simulink model "MATE_Pejovic_inverter"  (R2024b)
settings: Solver=FixedStepDiscrete  StartTime=0.0  StopTime=0.01  FixedStep=Ts  RelTol=1e-3
PostLoadFcn:
  | Ts=1e-6
InitFcn:
  | Ts=1e-6
libraries: fl_lib x29, nesl_utility x14, simetranss x4, batteryecm_lib x3
settings Model: ARTEMISmethode_block_infos=$$__separator__$$  Creator=Kyle Diller  LastModifiedBy=CD8435
settings SolverCC: MaxOrder=2  AlgebraicLoopSolver=TrustRegion
settings DataIOCC: SaveFormat=Array  SignalLoggingSaveFormat=ModelDataLogs  ReturnWorkspaceOutputs=off  SignalLoggingName=sigsOut
settings OptimizationCC: BlockReduction=off  BooleanDataType=off  ExpressionDepthLimit=2147483647  InitFltsAndDblsToZero=on  LifeSpan=inf
settings DebuggingCC: SaveWithParameterizedLinksMsg=none  UnderspecifiedInitializationDetection=Classic  MergeDetectMultiDrivingBlocksExec=none  SignalResolutionControl=TryResolveAllWithWarning  MultiTaskDSMMsg=warning  MultiTaskCondExecSysMsg=none  FcnCallInpInsideContextMsg=warning  UnconnectedInputMsg=warning  UnconnectedOutputMsg=warning  UnconnectedLineMsg=warning  AllowSymbolicDim=off  StateNameClashWarn=warning  SFUnexpectedBacktrackingDiag=warning  SFNoUnconditionalDefaultTransitionDiag=warning  SFExecutionAtInitializationDiag=none  ArithmeticOperatorsInVariantConditions=warning
settings HardwareCC: ProdBitPerPointer=32  ProdBitPerSizeT=32  ProdBitPerPtrDiffT=32  ProdLargestAtomicFloat=None  ProdIntDivRoundTo=Undefined  ProdEndianess=Unspecified  ProdWordSize=32  ProdHWDeviceType=32-bit Generic  TargetUnknown=on
settings ModelReferenceCC: EnableRefExpFcnMdlSchedulingChecks=on  PropagateSignalLabelsOutOfModel=off
settings SFSimCC: SimUseLocalCustomCode=off  CustomCodeUndefinedFunction=UseInterfaceOnly
settings RTWCC: TemplateMakefile=grt_unix.tmf  RTWUseLocalCustomCode=off  GPUComputeCapability=3.5
settings CodeAppCC: StateflowObjectComments=on
settings GRTTargetCC: TargetFcnLib=ansi_tfl_tmw.mat  TargetLangStandard=C89/C90 (ANSI)  CombineOutputUpdateFcns=off  GRTInterface=on
settings ConfigComp: CovMetricSettings=dw  CovSaveCumulativeToWorkspaceVar=on  CovSaveSingleToWorkspaceVar=on  CovExternalEMLEnable=off
settings SimscapeCC: SimscapeNormalizeSystem=off

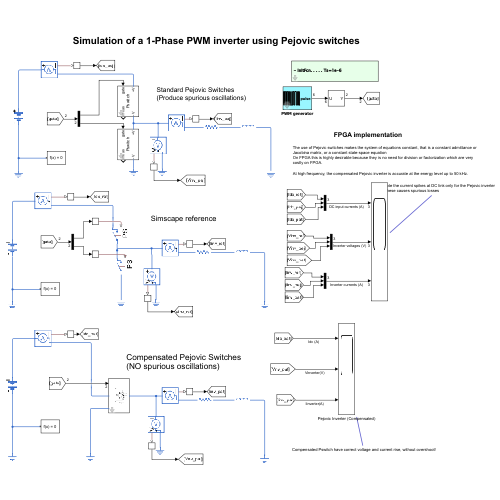
[thumbnail: Simulink's stored preview of the top-level diagram]
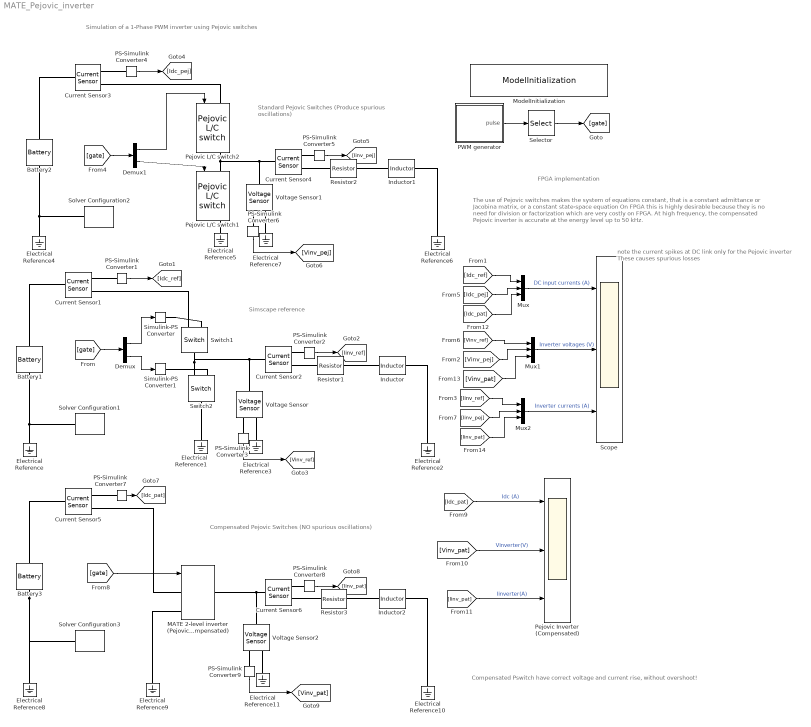
== system MATE_Pejovic_inverter ==
  note: The use of Pejovic switches makes the system of equations constant, that is a constant admittance or Jacobina matrix, or a constant state-space equation
      | On FPGA this is highly desirable because they is no need for division or factorization which are very costly on FPGA.
      |
      | At high frequency, the compensated Pejovic inverter is accurate at the energy level up to 50 kHz.
  note: FPGA implementation
  note: Simscape reference
  note: Standard Pejovic Switches
      | (Produce spurious oscillations)
  note: Compensated Pswitch have correct voltage and current rise, without overshoot!
  note: note the current spikes at DC link only for the Pejovic inverter
      | These causes spurious losses
  note: Simulation of a 1-Phase PWM inverter using Pejovic switches
  note: Compensated Pejovic Switches
      | (NO spurious oscillations)
  Battery1 : batteryecm_lib/Battery  Vnom=100 V  prm_dir=simscape.enum.battery.prm_dir.disabled  R1_dis=2 Ohm  R1_ch=2 Ohm  R1=0.5 Ohm  prm_AH=simscape.enum.battery.prm_AH.infinite  AH=50 A*hr  V1=11.5 V  AH1=25 A*hr  prm_R2=simscape.enum.battery.prm_R2.disabled  R2=2000 Ohm  Tmeas=298.15 K  charge_measurement_port=simscape.enum.battery.enable.no  prm_dyn=simscape.enum.battery.prm_dyn.off  Rp1=0.005 Ohm  tau1=30 s  Rp2=0.005 Ohm  tau2=30 s  Rp3=0.005 Ohm  tau3=30 s  Rp4=0.005 Ohm  tau4=30 s  Rp5=0.005 Ohm  tau5=30 s  prm_fade=simscape.enum.battery.prm_fade.disabled  N_fade=100  AH_fade=45 A*hr  R1_fade=2.02 Ohm  R1_ch_fade=2.02 Ohm  V1_fade=10.35 V  prm_age=simscape.enum.battery.prm_age.disabled  prm_age_OCV=simscape.enum.battery.prm_age_OCV.OCV  OCV_age=0.9  SOC_age=60  Tmeas_age=298.15 K  delta_time_age_vec=[0] d  temperature_age_vec=[273] K  OCV_scaling_age=2.2134e6  OCV_offset_age=1.632e6  temp_exp_age=0.515833569 V  t_exp_age=0.75  Vnom_T2=12 V  R1_T2=2.2 Ohm  R1_T2_dis=2.2 Ohm  R1_T2_ch=2.2 Ohm  V1_T2=11.4 V  R2_T2=2200 Ohm  Rp1_T2=0.005 Ohm  tau1_T2=30 s  Rp2_T2=0.005 Ohm  tau2_T2=30 s  Rp3_T2=0.005 Ohm  tau3_T2=30 s  Rp4_T2=0.005 Ohm  tau4_T2=30 s  Rp5_T2=0.005 Ohm  tau5_T2=30 s  Tmeas2=273.15 K  thermal_port=simscape.enum.thermaleffects.omit  thermal_mass=30000 J/K  i_specify=off  i_priority=None  i=0 A  i_nominal_specify=off  i_nominal_value=1  i_nominal_unit=A  v_specify=off  v_priority=None  v=0 V  v_nominal_specify=off  v_nominal_value=1  v_nominal_unit=V  charge_specify=off  charge_priority=High  charge=50 A*hr  charge_nominal_specify=off  charge_nominal_value=1  charge_nominal_unit=A*hr  num_cycles_specify=off  num_cycles_priority=High  num_cycles=0  num_cycles_nominal_specify=off  num_cycles_nominal_value=1  num_cycles_nominal_unit=1  temperature_specify=off  temperature_priority=High  temperature=298.15 K  temperature_nominal_specify=off  temperature_nominal_value=1  temperature_nominal_unit=K
  Battery2 : batteryecm_lib/Battery  Vnom=100 V  prm_dir=simscape.enum.battery.prm_dir.disabled  R1_dis=2 Ohm  R1_ch=2 Ohm  R1=0.5 Ohm  prm_AH=simscape.enum.battery.prm_AH.infinite  AH=50 A*hr  V1=11.5 V  AH1=25 A*hr  prm_R2=simscape.enum.battery.prm_R2.disabled  R2=2000 Ohm  Tmeas=298.15 K  charge_measurement_port=simscape.enum.battery.enable.no  prm_dyn=simscape.enum.battery.prm_dyn.off  Rp1=0.005 Ohm  tau1=30 s  Rp2=0.005 Ohm  tau2=30 s  Rp3=0.005 Ohm  tau3=30 s  Rp4=0.005 Ohm  tau4=30 s  Rp5=0.005 Ohm  tau5=30 s  prm_fade=simscape.enum.battery.prm_fade.disabled  N_fade=100  AH_fade=45 A*hr  R1_fade=2.02 Ohm  R1_ch_fade=2.02 Ohm  V1_fade=10.35 V  prm_age=simscape.enum.battery.prm_age.disabled  prm_age_OCV=simscape.enum.battery.prm_age_OCV.OCV  OCV_age=0.9  SOC_age=60  Tmeas_age=298.15 K  delta_time_age_vec=[0] d  temperature_age_vec=[273] K  OCV_scaling_age=2.2134e6  OCV_offset_age=1.632e6  temp_exp_age=0.515833569 V  t_exp_age=0.75  Vnom_T2=12 V  R1_T2=2.2 Ohm  R1_T2_dis=2.2 Ohm  R1_T2_ch=2.2 Ohm  V1_T2=11.4 V  R2_T2=2200 Ohm  Rp1_T2=0.005 Ohm  tau1_T2=30 s  Rp2_T2=0.005 Ohm  tau2_T2=30 s  Rp3_T2=0.005 Ohm  tau3_T2=30 s  Rp4_T2=0.005 Ohm  tau4_T2=30 s  Rp5_T2=0.005 Ohm  tau5_T2=30 s  Tmeas2=273.15 K  thermal_port=simscape.enum.thermaleffects.omit  thermal_mass=30000 J/K  i_specify=off  i_priority=None  i=0 A  i_nominal_specify=off  i_nominal_value=1  i_nominal_unit=A  v_specify=off  v_priority=None  v=0 V  v_nominal_specify=off  v_nominal_value=1  v_nominal_unit=V  charge_specify=off  charge_priority=High  charge=50 A*hr  charge_nominal_specify=off  charge_nominal_value=1  charge_nominal_unit=A*hr  num_cycles_specify=off  num_cycles_priority=High  num_cycles=0  num_cycles_nominal_specify=off  num_cycles_nominal_value=1  num_cycles_nominal_unit=1  temperature_specify=off  temperature_priority=High  temperature=298.15 K  temperature_nominal_specify=off  temperature_nominal_value=1  temperature_nominal_unit=K
  Battery3 : batteryecm_lib/Battery  Vnom=100 V  prm_dir=simscape.enum.battery.prm_dir.disabled  R1_dis=2 Ohm  R1_ch=2 Ohm  R1=0.5 Ohm  prm_AH=simscape.enum.battery.prm_AH.infinite  AH=50 A*hr  V1=11.5 V  AH1=25 A*hr  prm_R2=simscape.enum.battery.prm_R2.disabled  R2=2000 Ohm  Tmeas=298.15 K  charge_measurement_port=simscape.enum.battery.enable.no  prm_dyn=simscape.enum.battery.prm_dyn.off  Rp1=0.005 Ohm  tau1=30 s  Rp2=0.005 Ohm  tau2=30 s  Rp3=0.005 Ohm  tau3=30 s  Rp4=0.005 Ohm  tau4=30 s  Rp5=0.005 Ohm  tau5=30 s  prm_fade=simscape.enum.battery.prm_fade.disabled  N_fade=100  AH_fade=45 A*hr  R1_fade=2.02 Ohm  R1_ch_fade=2.02 Ohm  V1_fade=10.35 V  prm_age=simscape.enum.battery.prm_age.disabled  prm_age_OCV=simscape.enum.battery.prm_age_OCV.OCV  OCV_age=0.9  SOC_age=60  Tmeas_age=298.15 K  delta_time_age_vec=[0] d  temperature_age_vec=[273] K  OCV_scaling_age=2.2134e6  OCV_offset_age=1.632e6  temp_exp_age=0.515833569 V  t_exp_age=0.75  Vnom_T2=12 V  R1_T2=2.2 Ohm  R1_T2_dis=2.2 Ohm  R1_T2_ch=2.2 Ohm  V1_T2=11.4 V  R2_T2=2200 Ohm  Rp1_T2=0.005 Ohm  tau1_T2=30 s  Rp2_T2=0.005 Ohm  tau2_T2=30 s  Rp3_T2=0.005 Ohm  tau3_T2=30 s  Rp4_T2=0.005 Ohm  tau4_T2=30 s  Rp5_T2=0.005 Ohm  tau5_T2=30 s  Tmeas2=273.15 K  thermal_port=simscape.enum.thermaleffects.omit  thermal_mass=30000 J/K  i_specify=off  i_priority=None  i=0 A  i_nominal_specify=off  i_nominal_value=1  i_nominal_unit=A  v_specify=off  v_priority=None  v=0 V  v_nominal_specify=off  v_nominal_value=1  v_nominal_unit=V  charge_specify=off  charge_priority=High  charge=50 A*hr  charge_nominal_specify=off  charge_nominal_value=1  charge_nominal_unit=A*hr  num_cycles_specify=off  num_cycles_priority=High  num_cycles=0  num_cycles_nominal_specify=off  num_cycles_nominal_value=1  num_cycles_nominal_unit=1  temperature_specify=off  temperature_priority=High  temperature=298.15 K  temperature_nominal_specify=off  temperature_nominal_value=1  temperature_nominal_unit=K
  Current Sensor{1..6} (6 alike) : fl_lib/Electrical/Electrical Sensors/Current Sensor
  Demux : Demux  Outputs=2
  Demux1 : Demux  Outputs=2
  Electrical Reference{,1..11} (12 alike) : fl_lib/Electrical/Electrical Elements/Electrical Reference
  Inductor : fl_lib/Electrical/Electrical Elements/Inductor  l=1e-4 H  r=0 Ohm  g=1e-9 1/Ohm  i_specify=off  i_priority=None  i=0 A  i_nominal_specify=off  i_nominal_value=1  i_nominal_unit=A  v_specify=off  v_priority=None  v=0 V  v_nominal_specify=off  v_nominal_value=1  v_nominal_unit=V  i_L_specify=off  i_L_priority=High  i_L=0 A  i_L_nominal_specify=off  i_L_nominal_value=1  i_L_nominal_unit=A
  Inductor1 : fl_lib/Electrical/Electrical Elements/Inductor  l=1e-4 H  r=0 Ohm  g=1e-9 1/Ohm  i_specify=off  i_priority=None  i=0 A  i_nominal_specify=off  i_nominal_value=1  i_nominal_unit=A  v_specify=off  v_priority=None  v=0 V  v_nominal_specify=off  v_nominal_value=1  v_nominal_unit=V  i_L_specify=off  i_L_priority=High  i_L=0 A  i_L_nominal_specify=off  i_L_nominal_value=1  i_L_nominal_unit=A
  Inductor2 : fl_lib/Electrical/Electrical Elements/Inductor  l=1e-4 H  r=0 Ohm  g=1e-9 1/Ohm  i_specify=off  i_priority=None  i=0 A  i_nominal_specify=off  i_nominal_value=1  i_nominal_unit=A  v_specify=off  v_priority=None  v=0 V  v_nominal_specify=off  v_nominal_value=1  v_nominal_unit=V  i_L_specify=off  i_L_priority=High  i_L=0 A  i_L_nominal_specify=off  i_L_nominal_value=1  i_L_nominal_unit=A
  MATE 2-level inverter (Pejovic Energy compensated) : simetranss/FPGA/MATE 2-level inverter (Pejovic Energy compensated)  Lon=1e-6  Ts=Ts
  ModelInitialization : simetranss/Usefulls/ModelInitialization  InitFcnX=Ts=1e-6  prel=off  posl=on  inif=on  strf=off
  Mux : Mux  Inputs=3
  Mux1 : Mux  Inputs=3
  Mux2 : Mux  Inputs=3
  PS-Simulink Converter{1..9} (9 alike) : nesl_utility/PS-Simulink Converter  PhysicalDomain=network_engine_domain  SubClassName=ps_output  LeftPortType=input  RightPortType=output  PseudoPeriodic=off  Frequencies=[]  VectorFormat=inherit  Unit=inherit  AffineConversion=off
  PWM generator : Subsystem  Tag=RTEcontrol_s38shd7k88  mask(3-phase Discrete PWM Generator){Fc=1080, Ts=Ts, mIndex=0.6, Freq=60, Phase=0}
      mask prompts: Fc "Carrier frequency (Hz):"; Ts "Sample time:"; mIndex "Modulation index  (0<m<1) :"; Freq "Frequency of output voltage (Hz)"; Phase "Phase of output voltage (degrees)"
      mask help: This block generates pulses for 3-phase carrier-based PWM (Pulse Width Modulation), self-commutated IGBTs,GTOs or FETs bridges in Simscape.
      mask init:
      | if Freq==0
      |     Phase=90;
      | end
      |     Internal_Phase=[0 -2*pi/3 2*pi/3];
      |     Signal_PortWidth=3;
      |     Select1_Elements=[1 4 2 5 3 6];
      |     Select1_PortWidth=6;
      |    Select3_Elements=[1 2 3 4 5 6];
      |    Select3_PortWidth=12;
      mask Display: plot(0,0,100,100,[60,57,57,56,56,53,53,50,50,47,47,41,41,38,38,35,35,32,32,31,31,25,25,24,24,22,22,19,19,16,16,11,11,8,8,5,5,3,3,2,2,0],[20,20,80,80,20,20,80,80,20,20,80,80,20,20,80,80,20,20,80,80,20,20,80,80,20,20,80,80,20,20,80,80,20,20,80,80,20,20,80,80,20,20])
  Pejovic Inverter (Compensated) : Scope  NumInputPorts=3
  Pejovic L/C switch1 : simetranss/FPGA/Pejovic L//C switch  Lon=1e-6  Ts=Ts
  Pejovic L/C switch2 : simetranss/FPGA/Pejovic L//C switch  Lon=1e-6  Ts=Ts
  Resistor1 : fl_lib/Electrical/Electrical Elements/Resistor  R=9.5 Ohm  i_specify=off  i_priority=None  i=0 A  i_nominal_specify=off  i_nominal_value=1  i_nominal_unit=A  v_specify=off  v_priority=None  v=0 V  v_nominal_specify=off  v_nominal_value=1  v_nominal_unit=V
  Resistor2 : fl_lib/Electrical/Electrical Elements/Resistor  R=9.5 Ohm  i_specify=off  i_priority=None  i=0 A  i_nominal_specify=off  i_nominal_value=1  i_nominal_unit=A  v_specify=off  v_priority=None  v=0 V  v_nominal_specify=off  v_nominal_value=1  v_nominal_unit=V
  Resistor3 : fl_lib/Electrical/Electrical Elements/Resistor  R=9.5 Ohm  i_specify=off  i_priority=None  i=0 A  i_nominal_specify=off  i_nominal_value=1  i_nominal_unit=A  v_specify=off  v_priority=None  v=0 V  v_nominal_specify=off  v_nominal_value=1  v_nominal_unit=V
  Scope : Scope  NumInputPorts=3
  Selector : Selector  InputPortWidth=6  IndexOptions=Index vector (dialog)  Indices=[1 2]  OutputSizes=1
  Simulink-PS Converter : nesl_utility/Simulink-PS Converter  PhysicalDomain=network_engine_domain  SubClassName=ps_input  LeftPortType=input  RightPortType=output  PseudoPeriodic=off  Frequencies=[]  NoiseDistribution=none  NoiseParameters=[]  Unit=1  AffineConversion=off  FilteringAndDerivatives=provide  SimscapeFilterOrder=1  InputFilterTimeConstant=0.001  UdotUserProvided=0
  Simulink-PS Converter1 : nesl_utility/Simulink-PS Converter  PhysicalDomain=network_engine_domain  SubClassName=ps_input  LeftPortType=input  RightPortType=output  PseudoPeriodic=off  Frequencies=[]  NoiseDistribution=none  NoiseParameters=[]  Unit=1  AffineConversion=off  FilteringAndDerivatives=provide  SimscapeFilterOrder=1  InputFilterTimeConstant=0.001  UdotUserProvided=0
  Solver Configuration1 : nesl_utility/Solver Configuration  PhysicalDomain=network_engine_domain  SubClassName=solver  LeftPortType=input  RightPortType=generic  Tones=[]  Harmonics=[]  SimulateNoise=off  Profile=off  UseLocalSampling=off  EnableSwitchedLinearOptims=on  FrequencyDomain=off  UseCCode=off  RelTol=0.001  AbsTol=0.001  MinStep=1e-09  ToWorkspace=off  RevertToSquareIcSolve=off  NumHomotopyIterations=100  PhasorMode=off  PhasorModeNumHarmonics=1  ConsistencySolver=NEWTON_XTOL_AFTER_FTOL  IndexReductionMethod=DerivativeReplacement  DoDC=off  ResidualTolerance=1e-09  ConsistencyTolSource=GLOBAL  ConsistencyAbsTol=0.001  ConsistencyRelTol=0.001  ConsistencyTolFactor=0.001  UseLocalSolver=on  LocalSolverChoice=NE_PARTITIONING_ADVANCER  ResolveIndetEquations=on  FunctionEvalNumThread=1  LocalSolverSampleTime=Ts  DoFixedCost=on  MaxNonlinIter=1  MaxModeIter=2  ComputeImpulses=off  ImpulseIterations=2  LinearAlgebra=auto  LinearAlgebraNumThread=0  EquationFormulation=NE_TIME_EF  DelaysMemoryBudget=1024  AutomaticFiltering=on  FilteringTimeConstant=0.001  PartitionStorageMethod=AS_NEEDED  PartitionMemoryBudget=1024  PartitionMethod=ROBUST  MultibodyUseLocalSolver=off  MultibodyLocalSolverChoice=ODE1  MultibodyLocalSolverSampleTime=0.001
  Solver Configuration2 : nesl_utility/Solver Configuration  PhysicalDomain=network_engine_domain  SubClassName=solver  LeftPortType=input  RightPortType=generic  Tones=[]  Harmonics=[]  SimulateNoise=off  Profile=off  UseLocalSampling=off  EnableSwitchedLinearOptims=on  FrequencyDomain=off  UseCCode=off  RelTol=0.001  AbsTol=0.001  MinStep=1e-09  ToWorkspace=off  RevertToSquareIcSolve=off  NumHomotopyIterations=100  PhasorMode=off  PhasorModeNumHarmonics=1  ConsistencySolver=NEWTON_XTOL_AFTER_FTOL  IndexReductionMethod=DerivativeReplacement  DoDC=off  ResidualTolerance=1e-09  ConsistencyTolSource=GLOBAL  ConsistencyAbsTol=0.001  ConsistencyRelTol=0.001  ConsistencyTolFactor=0.001  UseLocalSolver=on  LocalSolverChoice=NE_BACKWARD_EULER_ADVANCER  ResolveIndetEquations=on  FunctionEvalNumThread=1  LocalSolverSampleTime=Ts  DoFixedCost=on  MaxNonlinIter=1  MaxModeIter=2  ComputeImpulses=off  ImpulseIterations=2  LinearAlgebra=auto  LinearAlgebraNumThread=0  EquationFormulation=NE_TIME_EF  DelaysMemoryBudget=1024  AutomaticFiltering=on  FilteringTimeConstant=0.001  PartitionStorageMethod=AS_NEEDED  PartitionMemoryBudget=1024  PartitionMethod=ROBUST  MultibodyUseLocalSolver=off  MultibodyLocalSolverChoice=ODE1  MultibodyLocalSolverSampleTime=0.001
  Solver Configuration3 : nesl_utility/Solver Configuration  PhysicalDomain=network_engine_domain  SubClassName=solver  LeftPortType=input  RightPortType=generic  Tones=[]  Harmonics=[]  SimulateNoise=off  Profile=off  UseLocalSampling=off  EnableSwitchedLinearOptims=on  FrequencyDomain=off  UseCCode=off  RelTol=0.001  AbsTol=0.001  MinStep=1e-09  ToWorkspace=off  RevertToSquareIcSolve=off  NumHomotopyIterations=100  PhasorMode=off  PhasorModeNumHarmonics=1  ConsistencySolver=NEWTON_XTOL_AFTER_FTOL  IndexReductionMethod=DerivativeReplacement  DoDC=off  ResidualTolerance=1e-09  ConsistencyTolSource=GLOBAL  ConsistencyAbsTol=0.001  ConsistencyRelTol=0.001  ConsistencyTolFactor=0.001  UseLocalSolver=on  LocalSolverChoice=NE_BACKWARD_EULER_ADVANCER  ResolveIndetEquations=on  FunctionEvalNumThread=1  LocalSolverSampleTime=Ts  DoFixedCost=on  MaxNonlinIter=1  MaxModeIter=2  ComputeImpulses=off  ImpulseIterations=2  LinearAlgebra=auto  LinearAlgebraNumThread=0  EquationFormulation=NE_TIME_EF  DelaysMemoryBudget=1024  AutomaticFiltering=on  FilteringTimeConstant=0.001  PartitionStorageMethod=AS_NEEDED  PartitionMemoryBudget=1024  PartitionMethod=ROBUST  MultibodyUseLocalSolver=off  MultibodyLocalSolverChoice=ODE1  MultibodyLocalSolverSampleTime=0.001
  Switch1 : fl_lib/Electrical/Electrical Elements/Switch  R_closed=0.001 Ohm  G_open=1e-8 1/Ohm  Threshold=0.5  i_specify=off  i_priority=None  i=0 A  i_nominal_specify=off  i_nominal_value=1  i_nominal_unit=A  v_specify=off  v_priority=None  v=0 V  v_nominal_specify=off  v_nominal_value=1  v_nominal_unit=V
  Switch2 : fl_lib/Electrical/Electrical Elements/Switch  R_closed=0.001 Ohm  G_open=1e-8 1/Ohm  Threshold=0.5  i_specify=off  i_priority=None  i=0 A  i_nominal_specify=off  i_nominal_value=1  i_nominal_unit=A  v_specify=off  v_priority=None  v=0 V  v_nominal_specify=off  v_nominal_value=1  v_nominal_unit=V
  Voltage Sensor : fl_lib/Electrical/Electrical Sensors/Voltage Sensor
  Voltage Sensor1 : fl_lib/Electrical/Electrical Sensors/Voltage Sensor
  Voltage Sensor2 : fl_lib/Electrical/Electrical Sensors/Voltage Sensor
  wires:
  PWM generator/1(pulse) -> Selector/1
  Demux/1 -> Simulink-PS Converter/1
  Demux/2 -> Simulink-PS Converter1/1
  Selector/1 -> [gate]
  [gate] -> Demux/1
  PS-Simulink Converter1/1 -> [Idc_ref]
  PS-Simulink Converter2/1 -> [Iinv_ref]
  PS-Simulink Converter3/1 -> [Vinv_ref]
  PS-Simulink Converter6/1 -> [Vinv_pej]
  PS-Simulink Converter5/1 -> [Iinv_pej]
  PS-Simulink Converter4/1 -> [Idc_pej]
  [gate] -> Demux1/1
  Demux1/1 -> Pejovic L/C switch2/1
  Demux1/2 -> Pejovic L/C switch1/1
  Mux/1 -> Scope/1  "DC input currents (A)"
  [Idc_pej] -> Mux/2
  [Idc_ref] -> Mux/1
  [Vinv_pej] -> Mux1/2
  Mux1/1 -> Scope/2  "Inverter voltages (V)"
  [Vinv_ref] -> Mux1/1
  Mux2/1 -> Scope/3  "Inverter currents (A)"
  [Iinv_ref] -> Mux2/1
  [Iinv_pej] -> Mux2/2
  PS-Simulink Converter7/1 -> [Idc_pat]
  PS-Simulink Converter8/1 -> [Iinv_pat]
  PS-Simulink Converter9/1 -> [Vinv_pat]
  [Idc_pat] -> Pejovic Inverter (Compensated)/1  "Idc (A)"
  [Vinv_pat] -> Pejovic Inverter (Compensated)/2  "Vinverter(V)"
  [Iinv_pat] -> Pejovic Inverter (Compensated)/3  "Iinverter(A)"
  [Idc_pat] -> Mux/3
  [Vinv_pat] -> Mux1/3
  [Iinv_pat] -> Mux2/3
  [gate] -> MATE 2-level inverter (Pejovic Energy compensated)/1
  connections:
  Electrical Reference/LConn1 -- Solver Configuration1/RConn1 -- Battery1/RConn1
  Battery1/LConn1 -- Current Sensor1/LConn1
  Current Sensor1/RConn2 -- Switch1/RConn2
  Switch2/RConn2 -- Voltage Sensor/LConn1 -- Current Sensor2/LConn1 -- Switch1/LConn1
  Electrical Reference1/LConn1 -- Switch2/LConn1
  Inductor/LConn1 -- Resistor1/RConn1
  Inductor/RConn1 -- Electrical Reference2/LConn1
  Current Sensor2/RConn2 -- Resistor1/LConn1
  PS-Simulink Converter1/LConn1 -- Current Sensor1/RConn1
  PS-Simulink Converter2/LConn1 -- Current Sensor2/RConn1
  Electrical Reference3/LConn1 -- Voltage Sensor/RConn2
  PS-Simulink Converter3/LConn1 -- Voltage Sensor/RConn1
  Simulink-PS Converter/RConn1 -- Switch1/RConn1
  Simulink-PS Converter1/RConn1 -- Switch2/RConn1
  Electrical Reference4/LConn1 -- Battery2/RConn1 -- Solver Configuration2/RConn1
  PS-Simulink Converter6/LConn1 -- Voltage Sensor1/RConn1
  Electrical Reference7/LConn1 -- Voltage Sensor1/RConn2
  PS-Simulink Converter5/LConn1 -- Current Sensor4/RConn1
  PS-Simulink Converter4/LConn1 -- Current Sensor3/RConn1
  Inductor1/LConn1 -- Resistor2/RConn1
  Current Sensor4/RConn2 -- Resistor2/LConn1
  Inductor1/RConn1 -- Electrical Reference6/LConn1
  Battery2/LConn1 -- Current Sensor3/LConn1
  Pejovic L/C switch2/LConn1 -- Current Sensor3/RConn2
  Current Sensor4/LConn1 -- Pejovic L/C switch1/LConn1 -- Pejovic L/C switch2/RConn1 -- Voltage Sensor1/LConn1
  Pejovic L/C switch1/RConn1 -- Electrical Reference5/LConn1
  Battery3/RConn1 -- Electrical Reference8/LConn1 -- Solver Configuration3/RConn1
  Current Sensor6/LConn1 -- MATE 2-level inverter (Pejovic Energy compensated)/RConn1 -- Voltage Sensor2/LConn1
  Battery3/LConn1 -- Current Sensor5/LConn1
  Inductor2/RConn1 -- Electrical Reference10/LConn1
  Current Sensor6/RConn2 -- Resistor3/LConn1
  Electrical Reference11/LConn1 -- Voltage Sensor2/RConn2
  PS-Simulink Converter8/LConn1 -- Current Sensor6/RConn1
  PS-Simulink Converter7/LConn1 -- Current Sensor5/RConn1
  PS-Simulink Converter9/LConn1 -- Voltage Sensor2/RConn1
  Inductor2/LConn1 -- Resistor3/RConn1
  MATE 2-level inverter (Pejovic Energy compensated)/LConn1 -- Current Sensor5/RConn2
  MATE 2-level inverter (Pejovic Energy compensated)/LConn2 -- Electrical Reference9/LConn1

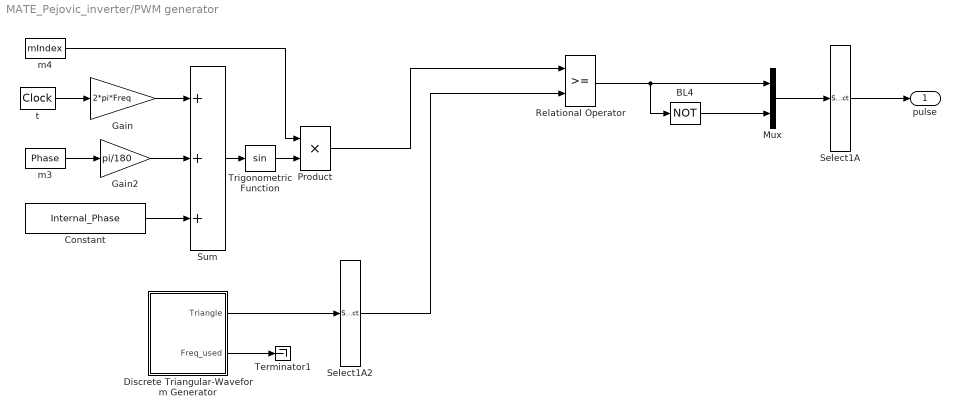
== system MATE_Pejovic_inverter/PWM generator ==
  BL4 : Logic  Operator=NOT  Inputs=1
  Constant : Constant  Value=Internal_Phase
  Discrete Triangular-Waveform Generator : Subsystem  mask(Discrete Triangular-Waveform  Generator){Freq=Fc, Vpeak=1, Ts=Ts}
      mask prompts: Freq "Frequency (Hz):"; Vpeak "Peak value:"; Ts "Sample time:"
      mask init:
      | NumberStepsRounded=round(1/Freq/Ts);
      | % Selection of an even number of steps
      | if mod(NumberStepsRounded,2)==0
      |    NumberSteps=NumberStepsRounded;
      | else
      |    NumberSteps=NumberStepsRounded+1;
      | end
      | Freq_used=1/(NumberSteps*Ts);
  Gain : Gain  Gain=2*pi*Freq  SaturateOnIntegerOverflow=on  OutDataTypeStr=Inherit: Same as input  ParamDataTypeStr=Inherit: Same as input
  Gain2 : Gain  Gain=pi/180  SaturateOnIntegerOverflow=on  OutDataTypeStr=Inherit: Same as input  ParamDataTypeStr=Inherit: Same as input
  Mux : Mux  Inputs=2
  Product : Product  InputSameDT=on  SaturateOnIntegerOverflow=on  OutDataTypeStr=Inherit: Same as first input
  Relational Operator : RelationalOperator
  Select1A : Selector  InputPortWidth=6  IndexOptions=Index vector (dialog)  Indices=Select1_Elements  OutputSizes=1
  Select1A2 : Selector  InputPortWidth=1  IndexOptions=Index vector (dialog)  Indices=[1 1 1]  OutputSizes=1
  Sum : Sum  Inputs=+++  InputSameDT=on  SaturateOnIntegerOverflow=on  OutDataTypeStr=Inherit: Same as first input
  Terminator1 : Terminator
  Trigonometric Function : Trigonometry
  m3 : Constant  Value=Phase
  m4 : Constant  Value=mIndex
  t : DigitalClock  SampleTime=Ts
  pulse : Outport  VectorParamsAs1DForOutWhenUnconnected=off
  wires:
  Select1A2/1 -> Relational Operator/2
  Select1A/1 -> pulse/1
  Discrete Triangular-Waveform Generator/1(Triangle) -> Select1A2/1
  Mux/1 -> Select1A/1
  BL4/1 -> Mux/2
  Discrete Triangular-Waveform Generator/2(Freq_used) -> Terminator1/1
  Product/1 -> Relational Operator/1
  Trigonometric Function/1 -> Product/2
  Sum/1 -> Trigonometric Function/1
  m4/1 -> Product/1
  Constant/1 -> Sum/3
  m3/1 -> Gain2/1
  Gain2/1 -> Sum/2
  Gain/1 -> Sum/1
  t/1 -> Gain/1
  Relational Operator/1 -> BL4/1, Mux/1

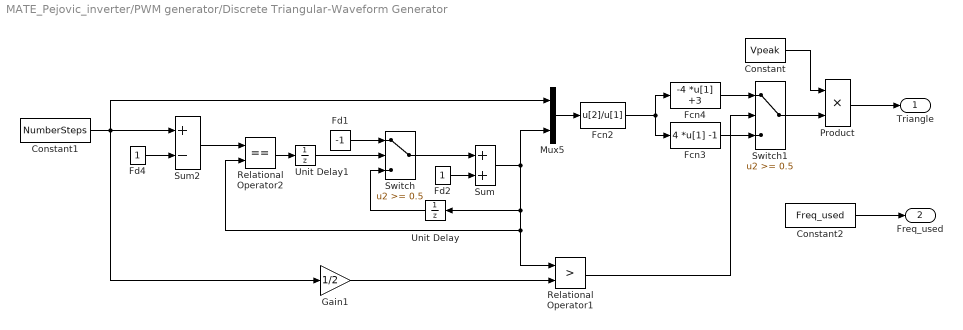
== system MATE_Pejovic_inverter/PWM generator/Discrete Triangular-Waveform Generator ==
  Constant : Constant  Value=Vpeak
  Constant1 : Constant  Value=NumberSteps
  Constant2 : Constant  Value=Freq_used
  Fcn2 : Fcn  Expr=u[2]/u[1]
  Fcn3 : Fcn  Expr=4 *u[1] -1
  Fcn4 : Fcn  Expr=-4 *u[1] +3
  Fd1 : Constant  Value=-1
  Fd2 : Constant
  Fd4 : Constant
  Gain1 : Gain  Gain=1/2  SaturateOnIntegerOverflow=on  OutDataTypeStr=Inherit: Same as input  ParamDataTypeStr=Inherit: Same as input
  Mux5 : Mux  Inputs=2
  Product : Product  InputSameDT=on  SaturateOnIntegerOverflow=on  OutDataTypeStr=Inherit: Same as first input
  Relational Operator1 : RelationalOperator  Operator=>
  Relational Operator2 : RelationalOperator  Operator===
  Sum : Sum  InputSameDT=on  SaturateOnIntegerOverflow=on  OutDataTypeStr=Inherit: Same as first input
  Sum2 : Sum  Inputs=+-  InputSameDT=on  SaturateOnIntegerOverflow=on  OutDataTypeStr=Inherit: Same as first input
  Switch : Switch  Threshold=0.5
  Switch1 : Switch  Threshold=0.5
  Unit Delay : UnitDelay  SampleTime=Ts  HasFrameUpgradeWarning=on
  Unit Delay1 : UnitDelay  SampleTime=Ts  HasFrameUpgradeWarning=on
  Triangle : Outport  InitialOutput=0  VectorParamsAs1DForOutWhenUnconnected=off
  Freq_used : Outport  Port=2  InitialOutput=0  VectorParamsAs1DForOutWhenUnconnected=off
  wires:
  Product/1 -> Triangle/1
  Switch1/1 -> Product/2
  Constant/1 -> Product/1
  Fd4/1 -> Sum2/2
  Switch/1 -> Sum/1
  Fd2/1 -> Sum/2
  Fd1/1 -> Switch/1
  Unit Delay/1 -> Switch/3
  Unit Delay1/1 -> Switch/2
  Relational Operator2/1 -> Unit Delay1/1
  Sum2/1 -> Relational Operator2/1
  Constant1/1 -> Sum2/1, Mux5/1, Gain1/1
  Sum/1 -> Unit Delay/1, Relational Operator2/2, Relational Operator1/1, Mux5/2
  Fcn2/1 -> Fcn4/1, Fcn3/1
  Mux5/1 -> Fcn2/1
  Fcn4/1 -> Switch1/1
  Fcn3/1 -> Switch1/3
  Gain1/1 -> Relational Operator1/2
  Relational Operator1/1 -> Switch1/2
  Constant2/1 -> Freq_used/1
